simulink model "controller"  (R2020b)
settings: Solver=ode23  StartTime=0.0  StopTime=Tsim  RelTol=1e-3
values from neighbouring files (symbols this model uses):
  pg_traj = create_traj(state_list, Nsamples)    [ctrl_ds_setup.m]
undefined symbols (not defined in the file or in its folder): ctrl_cfg_rem
libraries: biped_lib x2
settings Model: Creator=isclab  LastModifiedBy=isclab
settings SFSimCC: MATLABDynamicMemAlloc=off

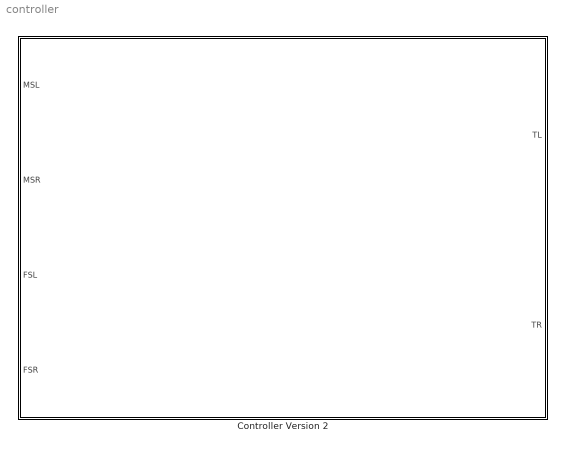
== system controller ==
  Controller Version 2 : Subsystem

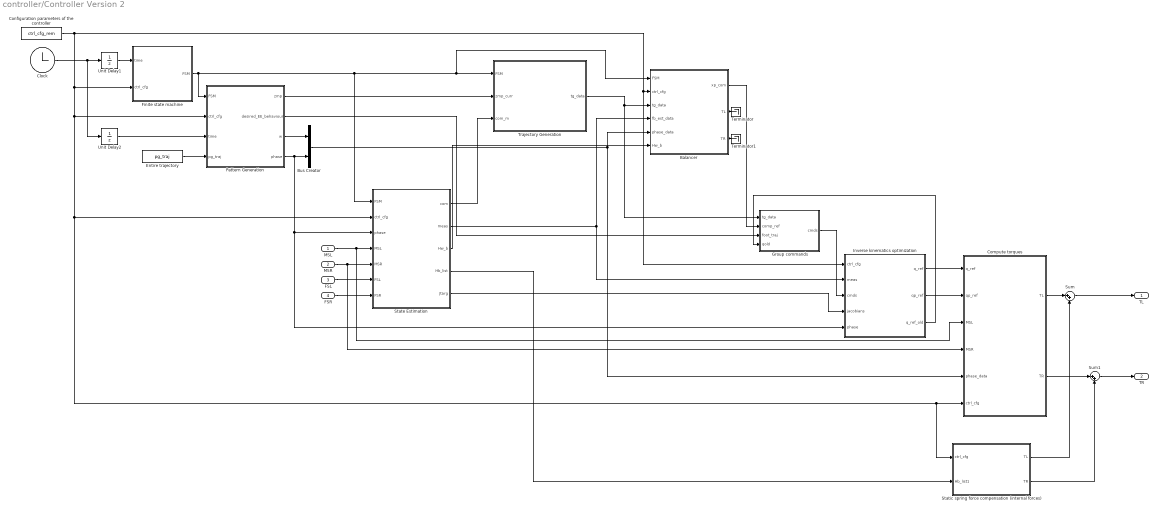
== system controller/Controller Version 2 ==
  MSL : Inport
  MSR : Inport  Port=2
  FSL : Inport  Port=3
  FSR : Inport  Port=4
  Balancer : MATLAB Function  TreatAsAtomicUnit=on
  Bus Creator : BusCreator  Inputs=2
  Clock : Clock
  Compute torques : Subsystem
  Configuration parameters of the controller : Constant  Value=ctrl_cfg_rem  OutDataTypeStr=Bus: ctrl_cfg_rem_bus  SampleTime=ctrl_cfg_rem.par.Ts
  Entire trajectory : Constant  Value=pg_traj  VectorParams1D=off  OutDataTypeStr=Bus: pg_traj_bus  SampleTime=ctrl_cfg_rem.par.Ts
  Finite state machine : MATLAB Function  TreatAsAtomicUnit=on
  Group commands : Subsystem
  Inverse kinematics optimization : Subsystem  Variant=on  mask{ik_opt=ctrl_cfg_rem.ik_opt, Ts=ctrl_cfg_rem.par.Ts}
      mask prompts: ik_opt "Ikine parameters"; Ts "Sampling time"
  Pattern Generation : Subsystem
  State Estimation : Subsystem  mask{fb_est=ctrl_cfg_rem.fb_est, Ts=ctrl_cfg_rem.par.Ts}
      mask prompts: fb_est "Floating base est. params"; Ts "Sampling time"
  Static spring force compensation (internal forces) : Subsystem
  Sum : Sum  Inputs=|++
  Sum1 : Sum  Inputs=|++
  Terminator : Terminator
  Terminator1 : Terminator
  Trajectory Generation : Subsystem  Variant=on  mask{tg=ctrl_cfg_rem.tg}
      mask prompts: tg "Preview controller parameters"
  Unit Delay1 : UnitDelay  SampleTime=ctrl_cfg_rem.par.Ts  HasFrameUpgradeWarning=on
  Unit Delay2 : UnitDelay  SampleTime=ctrl_cfg_rem.par.Ts  HasFrameUpgradeWarning=on
  TL : Outport
  TR : Outport  Port=2
  wires:
  Pattern Generation/1(zmp) -> Trajectory Generation/2(zmp_curr)
  Pattern Generation/4(phase) -> State Estimation/3(phase), Inverse kinematics optimization/5(phase), Bus Creator/2
  Unit Delay1/1 -> Finite state machine/1(time)
  Clock/1 -> Unit Delay2/1, Unit Delay1/1
  MSL/1 -> State Estimation/4(MSL), Compute torques/3(MSL)
  Entire trajectory/1 -> Pattern Generation/4(pg_traj)
  MSR/1 -> State Estimation/5(MSR), Compute torques/4(MSR)
  FSR/1 -> State Estimation/7(FSR)
  Configuration parameters of the controller/1 -> Inverse kinematics optimization/1(ctrl_cfg), Balancer/2(ctrl_cfg), Static spring force compensation (internal forces)/1(ctrl_cfg), Compute torques/6(ctrl_cfg), State Estimation/2(ctrl_cfg), Pattern Generation/2(ctrl_cfg), Finite state machine/2(ctrl_cfg)
  Finite state machine/1(FSM) -> Pattern Generation/1(FSM), State Estimation/1(FSM), Balancer/1(FSM), Trajectory Generation/1(FSM)
  Unit Delay2/1 -> Pattern Generation/3(time)
  FSL/1 -> State Estimation/6(FSL)
  Pattern Generation/3(w) -> Bus Creator/1
  Balancer/2(TL) -> Terminator/1
  Balancer/3(TR) -> Terminator1/1
  Bus Creator/1 -> Compute torques/5(phase_data), Balancer/5(phase_data)
  Inverse kinematics optimization/1(q_ref) -> Compute torques/1(q_ref)
  Inverse kinematics optimization/2(qp_ref) -> Compute torques/2(qp_ref)
  State Estimation/5(Jtarg) -> Inverse kinematics optimization/4(jacobians)
  Compute torques/1(TL) -> Sum/1
  Sum/1 -> TL/1
  Sum1/1 -> TR/1
  Compute torques/2(TR) -> Sum1/1
  State Estimation/4(Hb_list) -> Static spring force compensation (internal forces)/2(Hb_list1)
  Static spring force compensation (internal forces)/1(TL) -> Sum/2
  Static spring force compensation (internal forces)/2(TR) -> Sum1/2
  State Estimation/1(com) -> Trajectory Generation/3(com_m)
  State Estimation/2(meas) -> Inverse kinematics optimization/2(meas), Balancer/4(fb_est_data)
  Trajectory Generation/1(tg_data) -> Balancer/3(tg_data), Group commands/1(tg_data)
  Balancer/1(xp_com) -> Group commands/2(comp_ref)
  Pattern Generation/2(desired_EE_behaviour) -> Group commands/3(foot_traj)
  Group commands/1(cmds) -> Inverse kinematics optimization/3(cmds)
  State Estimation/3(Hw_b) -> Balancer/6(Hw_b)
  Inverse kinematics optimization/3(q_ref_old) -> Group commands/4(qold)

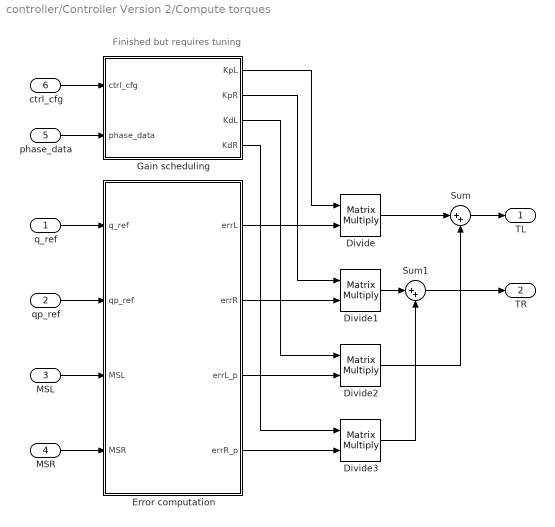
== system controller/Controller Version 2/Compute torques ==
  note: Finished but requires tuning
  q_ref : Inport
  qp_ref : Inport  Port=2
  MSL : Inport  Port=3
  MSR : Inport  Port=4
  phase_data : Inport  Port=5
  ctrl_cfg : Inport  Port=6
  Divide{,1..3} (4 alike) : Product  Inputs=**  Multiplication=Matrix(*)
  Error computation : MATLAB Function  TreatAsAtomicUnit=on
  Gain scheduling : MATLAB Function  TreatAsAtomicUnit=on
  Sum : Sum  Inputs=|++
  Sum1 : Sum  Inputs=|++
  TL : Outport
  TR : Outport  Port=2
  wires:
  phase_data/1 -> Gain scheduling/2(phase_data)
  MSL/1 -> Error computation/3(MSL)
  MSR/1 -> Error computation/4(MSR)
  qp_ref/1 -> Error computation/2(qp_ref)
  q_ref/1 -> Error computation/1(q_ref)
  Gain scheduling/1(KpL) -> Divide/1
  Error computation/1(errL) -> Divide/2
  Error computation/2(errR) -> Divide1/2
  Error computation/4(errR_p) -> Divide3/2
  Error computation/3(errL_p) -> Divide2/2
  Divide/1 -> Sum/1
  Divide2/1 -> Sum/2
  Sum/1 -> TL/1
  Divide1/1 -> Sum1/1
  Divide3/1 -> Sum1/2
  Sum1/1 -> TR/1
  ctrl_cfg/1 -> Gain scheduling/1(ctrl_cfg)
  Gain scheduling/2(KpR) -> Divide1/1
  Gain scheduling/3(KdL) -> Divide2/1
  Gain scheduling/4(KdR) -> Divide3/1

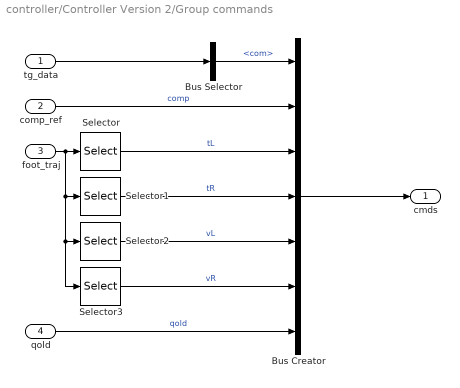
== system controller/Controller Version 2/Group commands ==
  tg_data : Inport
  comp_ref : Inport  Port=2
  foot_traj : Inport  Port=3
  qold : Inport  Port=4
  Bus Creator : BusCreator  Inputs=7
  Bus Selector : BusSelector  OutputSignals=com
  Selector : Selector  InputPortWidth=12  IndexOptions=Index vector (dialog)  Indices=[1:3]  OutputSizes=1
  Selector1 : Selector  InputPortWidth=12  IndexOptions=Index vector (dialog)  Indices=[4:6]  OutputSizes=1
  Selector2 : Selector  InputPortWidth=12  IndexOptions=Index vector (dialog)  Indices=[7:9]  OutputSizes=1
  Selector3 : Selector  InputPortWidth=12  IndexOptions=Index vector (dialog)  Indices=[10:12]  OutputSizes=1
  cmds : Outport
  wires:
  Bus Creator/1 -> cmds/1
  comp_ref/1 -> Bus Creator/2  "comp"
  tg_data/1 -> Bus Selector/1
  qold/1 -> Bus Creator/7  "qold"
  Bus Selector/1 -> Bus Creator/1  "<com>"
  foot_traj/1 -> Selector3/1, Selector2/1, Selector1/1, Selector/1
  Selector/1 -> Bus Creator/3  "tL"
  Selector1/1 -> Bus Creator/4  "tR"
  Selector2/1 -> Bus Creator/5  "vL"
  Selector3/1 -> Bus Creator/6  "vR"

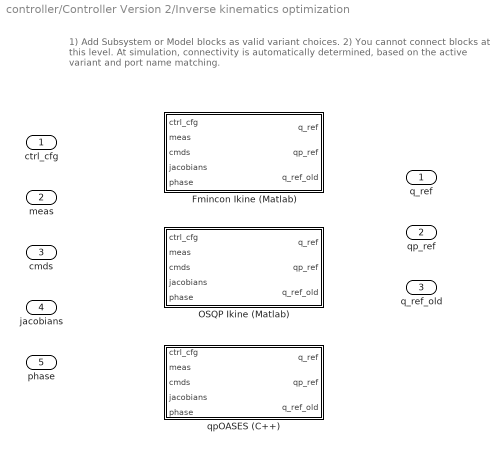
== system controller/Controller Version 2/Inverse kinematics optimization ==
  note: 1) Add Subsystem or Model blocks as valid variant choices.
      | 2) You cannot connect blocks at this level. At simulation, connectivity is automatically
      | determined, based on the active variant and port name matching.
  ctrl_cfg : Inport
  meas : Inport  Port=2
  cmds : Inport  Port=3
  jacobians : Inport  Port=4
  phase : Inport  Port=5
  Fmincon Ikine (Matlab) : Subsystem  VariantControl=VAR_IK ==1
  OSQP Ikine (Matlab) : Subsystem  VariantControl=VAR_IK ==2
  qpOASES (C++) : Subsystem  VariantControl=VAR_IK ==3
  q_ref : Outport
  qp_ref : Outport  Port=2
  q_ref_old : Outport  Port=3

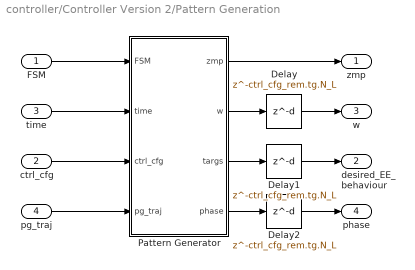
== system controller/Controller Version 2/Pattern Generation ==
  FSM : Inport
  ctrl_cfg : Inport  Port=2
  time : Inport  Port=3
  pg_traj : Inport  Port=4
  Delay : Delay  DelayLength=ctrl_cfg_rem.tg.N_L  InitialCondition=0  SampleTime=ctrl_cfg_rem.par.Ts
  Delay1 : Delay  DelayLength=ctrl_cfg_rem.tg.N_L  InitialCondition=0  SampleTime=ctrl_cfg_rem.par.Ts
  Delay2 : Delay  DelayLength=ctrl_cfg_rem.tg.N_L  InitialCondition=0  SampleTime=ctrl_cfg_rem.par.Ts
  Pattern Generator : MATLAB Function  TreatAsAtomicUnit=on
  zmp : Outport
  desired_EE_behaviour : Outport  Port=2
  w : Outport  Port=3
  phase : Outport  Port=4
  wires:
  Delay1/1 -> desired_EE_behaviour/1
  time/1 -> Pattern Generator/2(time)
  pg_traj/1 -> Pattern Generator/4(pg_traj)
  Delay/1 -> w/1
  FSM/1 -> Pattern Generator/1(FSM)
  Pattern Generator/1(zmp) -> zmp/1
  Pattern Generator/2(w) -> Delay/1
  ctrl_cfg/1 -> Pattern Generator/3(ctrl_cfg)
  Delay2/1 -> phase/1
  Pattern Generator/4(phase) -> Delay2/1
  Pattern Generator/3(targs) -> Delay1/1

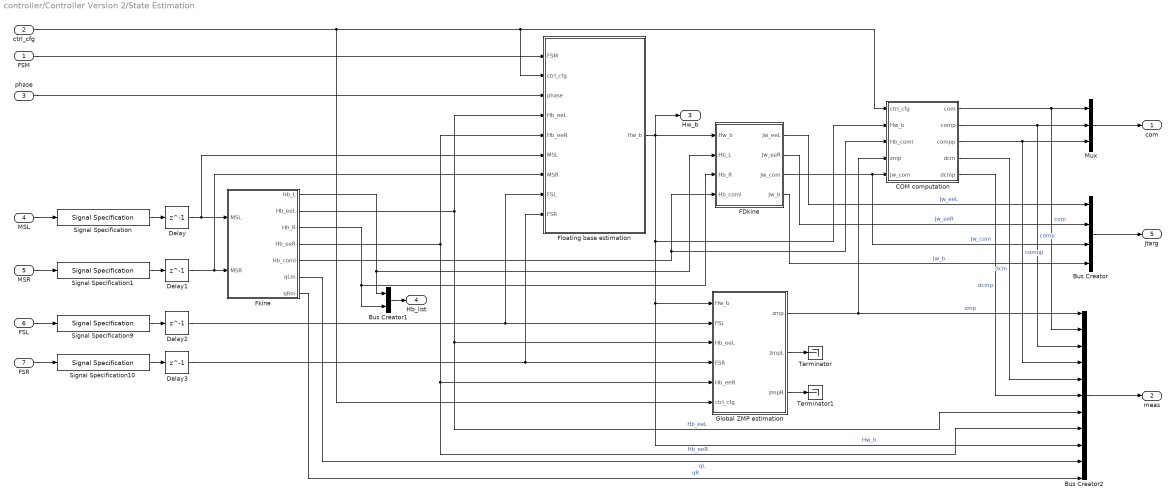
== system controller/Controller Version 2/State Estimation ==
  FSM : Inport
  ctrl_cfg : Inport  Port=2
  phase : Inport  Port=3
  MSL : Inport  Port=4
  MSR : Inport  Port=5
  FSL : Inport  Port=6
  FSR : Inport  Port=7
  Bus Creator : BusCreator  Inputs=4
  Bus Creator1 : BusCreator  Inputs=2
  Bus Creator2 : BusCreator  Inputs=11
  COM computation : MATLAB Function  TreatAsAtomicUnit=on
  Delay : Delay  DelayLength=1  InitialCondition=fb_est.init.MSL  SampleTime=Ts
  Delay1 : Delay  DelayLength=1  InitialCondition=fb_est.init.MSR  SampleTime=Ts
  Delay2 : Delay  DelayLength=1  InitialCondition=fb_est.init.FSL  SampleTime=Ts
  Delay3 : Delay  DelayLength=1  InitialCondition=fb_est.init.FSR  SampleTime=Ts
  FDkine : MATLAB Function  TreatAsAtomicUnit=on
  Fkine : MATLAB Function  TreatAsAtomicUnit=on
  Floating base estimation : MATLAB Function  TreatAsAtomicUnit=on
  Global ZMP estimation : MATLAB Function  TreatAsAtomicUnit=on
  Mux : Mux  Inputs=3
  Signal Specification : SignalSpecification  OutDataTypeStr=Bus: leg_str_bus
  Signal Specification1 : SignalSpecification  OutDataTypeStr=Bus: leg_str_bus
  Signal Specification10 : SignalSpecification  OutDataTypeStr=Bus: fs_str_bus
  Signal Specification9 : SignalSpecification  OutDataTypeStr=Bus: fs_str_bus
  Terminator : Terminator
  Terminator1 : Terminator
  com : Outport
  meas : Outport  Port=2
  Hw_b : Outport  Port=3
  Hb_list : Outport  Port=4
  Jtarg : Outport  Port=5
  wires:
  Signal Specification/1 -> Delay/1
  Signal Specification1/1 -> Delay1/1
  Signal Specification9/1 -> Delay2/1
  Signal Specification10/1 -> Delay3/1
  Delay2/1 -> Global ZMP estimation/2(FSL), Floating base estimation/8(FSL)
  Delay3/1 -> Global ZMP estimation/4(FSR), Floating base estimation/9(FSR)
  Fkine/1(Hb_L) -> Bus Creator1/1, FDkine/2(Hb_L)
  Fkine/3(Hb_R) -> Bus Creator1/2, FDkine/3(Hb_R)
  phase/1 -> Floating base estimation/3(phase)
  FSM/1 -> Floating base estimation/1(FSM)
  Floating base estimation/1(Hw_b) -> Hw_b/1, Bus Creator2/9, Global ZMP estimation/1(Hw_b), COM computation/2(Hw_b), FDkine/1(Hw_b)  "Hw_b"
  Fkine/5(Hb_comi) -> FDkine/4(Hb_comi), COM computation/3(Hb_comi)
  FDkine/3(Jw_com) -> COM computation/5(Jw_com), Bus Creator/3  "Jw_com"
  FDkine/1(Jw_eeL) -> Bus Creator/1  "Jw_eeL"
  FDkine/2(Jw_eeR) -> Bus Creator/2  "Jw_eeR"
  FDkine/4(Jw_b) -> Bus Creator/4  "Jw_b"
  Bus Creator/1 -> Jtarg/1
  ctrl_cfg/1 -> Global ZMP estimation/6(ctrl_cfg), COM computation/1(ctrl_cfg), Floating base estimation/2(ctrl_cfg)
  Global ZMP estimation/1(zmp) -> Bus Creator2/1, COM computation/4(zmp)  "zmp"
  Delay/1 -> Floating base estimation/6(MSL), Fkine/1(MSL)
  Delay1/1 -> Floating base estimation/7(MSR), Fkine/2(MSR)
  MSL/1 -> Signal Specification/1
  MSR/1 -> Signal Specification1/1
  FSL/1 -> Signal Specification9/1
  FSR/1 -> Signal Specification10/1
  Global ZMP estimation/2(zmpL) -> Terminator/1
  Global ZMP estimation/3(zmpR) -> Terminator1/1
  Bus Creator1/1 -> Hb_list/1
  COM computation/1(com) -> Mux/1, Bus Creator2/2  "com"
  COM computation/2(comp) -> Mux/2, Bus Creator2/3  "comp"
  COM computation/3(compp) -> Mux/3, Bus Creator2/4  "compp"
  COM computation/4(dcm) -> Bus Creator2/5  "dcm"
  COM computation/5(dcmp) -> Bus Creator2/6  "dcmp"
  Fkine/2(Hb_eeL) -> Floating base estimation/4(Hb_eeL), Global ZMP estimation/3(Hb_eeL), Bus Creator2/7  "Hb_eeL"
  Fkine/4(Hb_eeR) -> Floating base estimation/5(Hb_eeR), Global ZMP estimation/5(Hb_eeR), Bus Creator2/8  "Hb_eeR"
  Fkine/6(qLm) -> Bus Creator2/10  "qL"
  Fkine/7(qRm) -> Bus Creator2/11  "qR"
  Bus Creator2/1 -> meas/1
  Mux/1 -> com/1

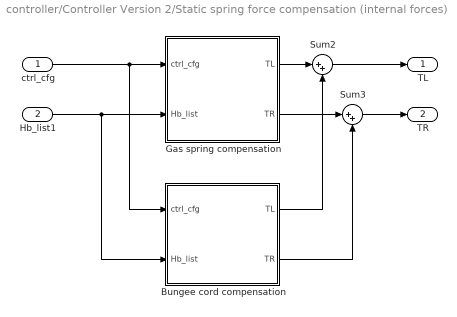
== system controller/Controller Version 2/Static spring force compensation (internal forces) ==
  ctrl_cfg : Inport
  Hb_list1 : Inport  Port=2
  Bungee cord compensation : MATLAB Function  TreatAsAtomicUnit=on
  Gas spring compensation : MATLAB Function  TreatAsAtomicUnit=on
  Sum2 : Sum  Inputs=|++
  Sum3 : Sum  Inputs=|++
  TL : Outport
  TR : Outport  Port=2
  wires:
  Bungee cord compensation/1(TL) -> Sum2/2
  Sum2/1 -> TL/1
  Sum3/1 -> TR/1
  Bungee cord compensation/2(TR) -> Sum3/2
  ctrl_cfg/1 -> Bungee cord compensation/1(ctrl_cfg), Gas spring compensation/1(ctrl_cfg)
  Hb_list1/1 -> Bungee cord compensation/2(Hb_list), Gas spring compensation/2(Hb_list)
  Gas spring compensation/1(TL) -> Sum2/1
  Gas spring compensation/2(TR) -> Sum3/1

== system controller/Controller Version 2/Trajectory Generation ==
  note: 1) Add Subsystem or Model blocks as valid variant choices.
      | 2) You cannot connect blocks at this level. At simulation, connectivity is automatically
      | determined, based on the active variant and port name matching.
  FSM : Inport
  zmp_curr : Inport  Port=2
  com_m : Inport  Port=3
  (C++ impl) : Subsystem  VariantControl=VAR_TG == 2
  Preview Controller (simulink impl) : Subsystem  VariantControl=VAR_TG == 1
  tg_data : Outport

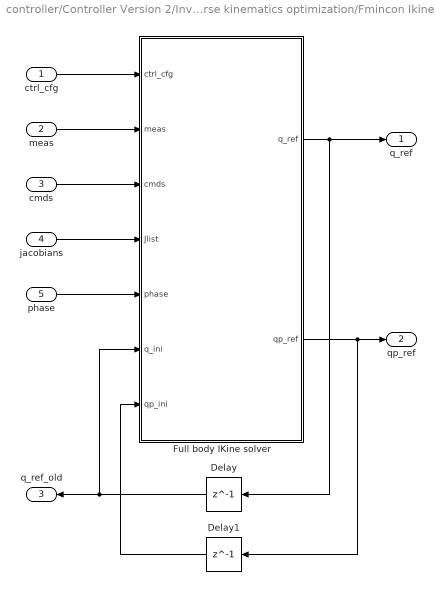
== system controller/Controller Version 2/Inverse kinematics optimization/Fmincon Ikine (Matlab) ==
  ctrl_cfg : Inport
  meas : Inport  Port=2
  cmds : Inport  Port=3
  jacobians : Inport  Port=4
  phase : Inport  Port=5
  Delay : Delay  DelayLength=1  InitialCondition=ik_opt.q_ini  SampleTime=Ts
  Delay1 : Delay  DelayLength=1  InitialCondition=ik_opt.qp_ini  SampleTime=Ts
  Full body IKine solver : MATLAB Function  TreatAsAtomicUnit=on
  q_ref : Outport
  qp_ref : Outport  Port=2
  q_ref_old : Outport  Port=3
  wires:
  Full body IKine solver/2(qp_ref) -> Delay1/1, qp_ref/1
  Full body IKine solver/1(q_ref) -> Delay/1, q_ref/1
  meas/1 -> Full body IKine solver/2(meas)
  cmds/1 -> Full body IKine solver/3(cmds)
  phase/1 -> Full body IKine solver/5(phase)
  jacobians/1 -> Full body IKine solver/4(Jlist)
  Delay/1 -> q_ref_old/1, Full body IKine solver/6(q_ini)
  Delay1/1 -> Full body IKine solver/7(qp_ini)
  ctrl_cfg/1 -> Full body IKine solver/1(ctrl_cfg)

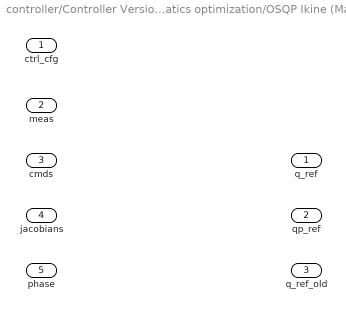
== system controller/Controller Version 2/Inverse kinematics optimization/OSQP Ikine (Matlab) ==
  ctrl_cfg : Inport
  meas : Inport  Port=2
  cmds : Inport  Port=3
  jacobians : Inport  Port=4
  phase : Inport  Port=5
  q_ref : Outport
  qp_ref : Outport  Port=2
  q_ref_old : Outport  Port=3

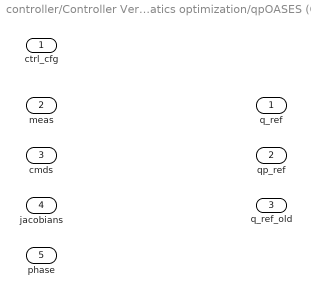
== system controller/Controller Version 2/Inverse kinematics optimization/qpOASES (C++) ==
  ctrl_cfg : Inport
  meas : Inport  Port=2
  cmds : Inport  Port=3
  jacobians : Inport  Port=4
  phase : Inport  Port=5
  q_ref : Outport
  qp_ref : Outport  Port=2
  q_ref_old : Outport  Port=3

== system controller/Controller Version 2/Trajectory Generation/(C++ impl) ==
  FSM : Inport
  zmp_curr : Inport  Port=2
  com_m : Inport  Port=3
  tg_data : Outport

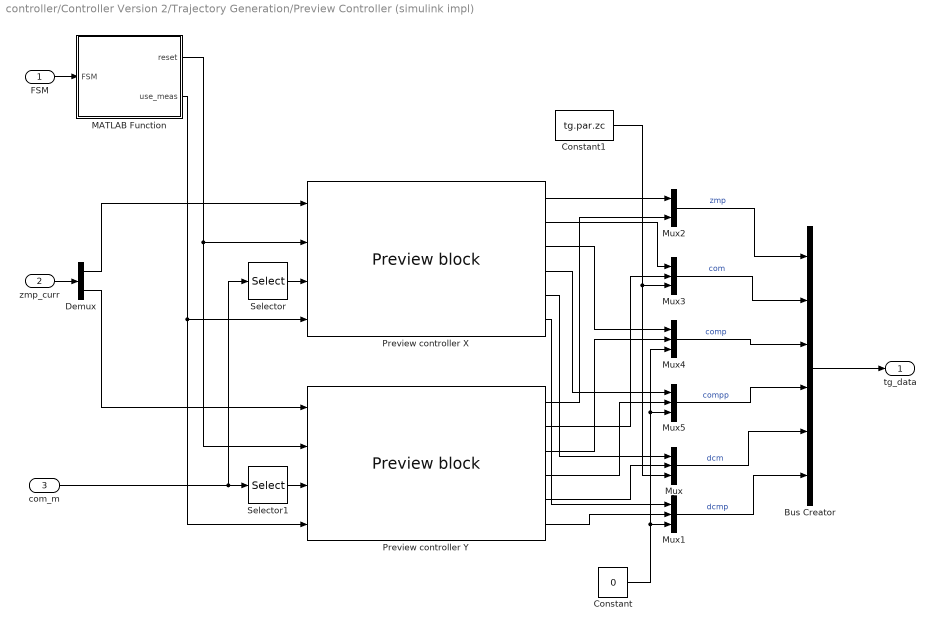
== system controller/Controller Version 2/Trajectory Generation/Preview Controller (simulink impl) ==
  FSM : Inport
  zmp_curr : Inport  Port=2
  com_m : Inport  Port=3
  Bus Creator : BusCreator  Inputs=6
  Constant : Constant  Value=0
  Constant1 : Constant  Value=tg.par.zc
  Demux : Demux  Outputs=2
  MATLAB Function : MATLAB Function  TreatAsAtomicUnit=on
  Mux{,1,3..5} (5 alike) : Mux  Inputs=3
  Mux2 : Mux  Inputs=2
  Preview controller X : biped_lib/Preview block  Pctrl=tg
  Preview controller Y : biped_lib/Preview block  Pctrl=tg
  Selector : Selector  InputPortWidth=6  IndexOptions=Index vector (dialog)  Indices=[1:3]  OutputSizes=1
  Selector1 : Selector  InputPortWidth=6  IndexOptions=Index vector (dialog)  Indices=[4:6]  OutputSizes=1
  tg_data : Outport
  wires:
  zmp_curr/1 -> Demux/1
  Demux/1 -> Preview controller X/1
  Demux/2 -> Preview controller Y/1
  com_m/1 -> Selector/1, Selector1/1
  Selector/1 -> Preview controller X/3
  Selector1/1 -> Preview controller Y/3
  FSM/1 -> MATLAB Function/1(FSM)
  MATLAB Function/1(reset) -> Preview controller X/2, Preview controller Y/2
  MATLAB Function/2(use_meas) -> Preview controller Y/4, Preview controller X/4
  Preview controller Y/5 -> Mux/2
  Preview controller Y/6 -> Mux1/2
  Preview controller X/5 -> Mux/1
  Preview controller X/6 -> Mux1/1
  Preview controller X/1 -> Mux2/1
  Preview controller Y/1 -> Mux2/2
  Mux2/1 -> Bus Creator/1  "zmp"
  Mux/1 -> Bus Creator/5  "dcm"
  Mux1/1 -> Bus Creator/6  "dcmp"
  Preview controller X/2 -> Mux3/1
  Preview controller Y/2 -> Mux3/2
  Mux3/1 -> Bus Creator/2  "com"
  Mux4/1 -> Bus Creator/3  "comp"
  Preview controller X/3 -> Mux4/1
  Preview controller Y/3 -> Mux4/2
  Mux5/1 -> Bus Creator/4  "compp"
  Preview controller X/4 -> Mux5/1
  Preview controller Y/4 -> Mux5/2
  Constant/1 -> Mux4/3, Mux5/3, Mux1/3
  Constant1/1 -> Mux3/3, Mux/3
  Bus Creator/1 -> tg_data/1

== matlab function controller/Controller Version 2/State Estimation/COM computation ==
  data: ctrl_cfg input; Hw_b input; Hb_comi input; zmp input; com output; comp output; compp output; dcm output; Jw_com input; dcmp output
function [com, comp, compp, dcm, dcmp] = fcn(ctrl_cfg, Hw_b, Hb_comi, zmp, Jw_com)
persistent init com_old comp_old compp_old;

fb_est = ctrl_cfg.fb_est;
Ts = fb_est.Ts;
omega = fb_est.omega;
mlist = fb_est.mlist;

% IIR filter parameters
alpha_cp = fb_est.alpha_cp;
alpha_cpp = fb_est.alpha_cpp;

if isempty(init)
    init = 1;
    com_old = fb_est.init.com; %prevents controller jumps
    comp_old = zeros(3,1);
    compp_old = zeros(3,1);
end

% compute com position in base frame
com_b = compute_com_pos(Hb_comi,mlist);

% get estimated com postion
com_w = Hw_b * [com_b;1];

% compute com outputs
com = com_w(1:3);
comp = alpha_cp*(com-com_old)/Ts + (1-alpha_cp)*comp_old;
compp = alpha_cpp*(comp-com_old)/Ts + (1-alpha_cpp)*compp_old;

% there is a possible way of computing the velocity using other data
% sources as well. Try it out if there is enough time.

% overwrite old values
com_old = com;
comp_old = comp;
compp_old = compp;

% compute dcm outputs
dcm = com + comp/omega;
dcmp = omega * (dcm - zmp);
dcmp_alt = comp + compp/omega; %alternative way of computing dcmp (lag version)

dcm_m = [dcm;dcmp];

== matlab function controller/Controller Version 2/State Estimation/Global ZMP estimation ==
  data: Hw_b input; zmp output; FSL input; Hb_eeL input; FSR input; Hb_eeR input; zmpL output; zmpR output; ctrl_cfg input
function [zmp,zmpL,zmpR] = fcn(Hw_b, FSL,Hb_eeL, FSR, Hb_eeR, ctrl_cfg)
    Hw_eeL = Hw_b * Hb_eeL;
    Hw_eeR = Hw_b * Hb_eeR;

    foot_data = ctrl_cfg.fb_est.foot_data;
    threshold_force = 1;
    simple_zmp = 0;
    [zmp,zmpL_full,zmpR_full] = compute_zmp_full(FSL, FSR, foot_data, Hw_eeL, Hw_eeR, threshold_force, simple_zmp); %computed zmp
    zmpL = zmpL_full.glo;
    zmpR = zmpR_full.glo;
end

== matlab function controller/Controller Version 2/Static spring force compensation (internal forces)/Bungee cord compensation ==
  data: ctrl_cfg input; Hb_list input; TL output; TR output
function [TL, TR] = fcn(ctrl_cfg, Hb_list)
    consts = ctrl_cfg.sf_comp.bc;
    HL = Hb_list.HL;
    HR = Hb_list.HR;
    [TL, TR] = bcordCompensTorques2(HL,HR,consts);
end

== matlab function controller/Controller Version 2/Compute torques/Gain scheduling ==
  data: ctrl_cfg input; phase_data input; KpL output; KpR output; KdL output; KdR output
function [KpL,KpR,KdL,KdR] = fcn(ctrl_cfg,phase_data)
    test_type = ctrl_cfg.fsm.test_type;
    w = phase_data.w;
    WshiftL = w(1);
    WshiftR = w(2);
    phase = phase_data.phase;
    [KpL, KpR, KdL, KdR] = get_gains2(test_type, phase, WshiftL, WshiftR);
end

== matlab function controller/Controller Version 2/Compute torques/Error computation ==
  data: q_ref input; qp_ref input; MSL input; errL output; MSR input; errR output; errL_p output; errR_p output
function [errL, errR, errL_p, errR_p] = fcn(q_ref, qp_ref, MSL, MSR)
% reference positions
qL_ref = q_ref(1:end/2);
qR_ref = q_ref(end/2+1:end);
% reference velocities
qLp_ref = qp_ref(1:end/2);
qRp_ref = qp_ref(end/2+1:end);

% measurement data
[LL,RL] = group_motor_data(MSL,MSR);
% measured positions
qL_m = LL.q;
qR_m = RL.q;
% measured velocities
qLp_m = LL.qp;
qRp_m = RL.qp;

% position errors
errL = qL_ref-qL_m;
errR = qR_ref-qR_m;

% velocity errors
errL_p = qLp_ref-qLp_m;
errR_p = qRp_ref-qRp_m;

== matlab function controller/Controller Version 2/Inverse kinematics optimization/Fmincon Ikine (Matlab)/Full body IKine solver ==
  data: ctrl_cfg input; meas input; q_ref output; cmds input; Jlist input; phase input; qp_ref output; q_ini input; qp_ini input
function [q_ref,qp_ref] = fcn(ctrl_cfg, meas, cmds, Jlist, phase, q_ini, qp_ini)
[q_ref,qp_ref] = ikine_step2(meas, cmds, q_ini, qp_ini, Jlist, ctrl_cfg);

== matlab function controller/Controller Version 2/Finite state machine ==
  data: time input; FSM output Bus: FSM_bus; ctrl_cfg input
function FSM = fcn(time, ctrl_cfg)

test_type = ctrl_cfg.fsm.test_type;
Tpause = ctrl_cfg.fsm.Tpause;

FSM = fsm_ctrl_struct;

% wait for the fb estimation to get the correct state
if time > Tpause
    FSM.bal.act = 1;
    if test_type ~= 0
        FSM.pg_act = 1;
        FSM.tg.act = 1;
    end
end

== matlab function controller/Controller Version 2/Pattern Generation/Pattern Generator ==
  data: FSM input; zmp output; time input; ctrl_cfg input; w output; targs output; phase output; pg_traj input
function [zmp,w,targs,phase]  = fcn(FSM, time, ctrl_cfg, pg_traj)
persistent t0;

traj = pg_traj;
Ts = ctrl_cfg.par.Ts;

if isempty(t0)
    t0 = time;
end

if ~FSM.pg_act
    %reset the time
    t0 = time;
    %output the zero values
    zmp = traj.zmp(:,1);
    w = traj.w(:,1);
    targs = [
        traj.foot.xL(:,1);
        traj.foot.xR(:,1);
        traj.foot.xLp(:,1);
        traj.foot.xRp(:,1);
    ];
    phase = traj.phase(1);
else
    t1 = time - t0;
    ii = round(t1/Ts);
    zmp = traj.zmp(:,ii);
    w = traj.w(:,ii);
    targs = [
        traj.foot.xL(:,ii);
        traj.foot.xR(:,ii);
        traj.foot.xLp(:,ii);
        traj.foot.xRp(:,ii);
    ];
    phase = traj.phase(ii);
end

== matlab function controller/Controller Version 2/Trajectory Generation/Preview Controller (simulink impl)/MATLAB Function ==
  data: FSM input; reset output; use_meas output
function [reset,use_meas] = fcn(FSM)
% flush buffer memory
if ~FSM.tg.act
    reset = 1;
else
    reset = 0;
end

% use feedback (measured COM)
if FSM.tg.use_fb
    use_meas = 1;
else
    use_meas = 0;
end

== matlab function controller/Controller Version 2/State Estimation/Fkine ==
  data: MSL input; Hb_L output; Hb_eeL output; MSR input; Hb_R output; Hb_eeR output; Hb_comi output; qLm output; qRm output
function [Hb_L, Hb_eeL, Hb_R, Hb_eeR, Hb_comi, qLm, qRm] = fcn(MSL,MSR)
    [LL,RL] = group_motor_data(MSL,MSR);
    qLm = LL.q;
    qRm = RL.q;
    [Hb_comi,Hb_L,Hb_R] = H_com_list(qLm,qRm);
    Hb_eeL = reshape(Hb_L(end,:,:),4,4);
    Hb_eeR = reshape(Hb_R(end,:,:),4,4);
end

== matlab function controller/Controller Version 2/State Estimation/Floating base estimation ==
  data: FSM input; ctrl_cfg input; phase input; Hb_eeL input; Hw_b output; Hb_eeR input; MSL input; MSR input; FSL input; FSR input
function Hw_b = fcn(FSM, ctrl_cfg, phase, Hb_eeL, Hb_eeR, MSL, MSR, FSL, FSR)
    persistent init Hw_L_corr Hw_R_corr;
    persistent quatLimu_old quatRimu_old;
    
    fb_est = ctrl_cfg.fb_est;
    cdf_data = fb_est.cdf_data;
    FootDataPmeas = fb_est.foot_data.fsen.Pmeas;
    
    %begin by not doing any compensation (IMU has no bias yet)
    if isempty(init)
        init = 1;
        %only executed at the init phase
        Hw_eeL = fb_est.init.Hw_eeL;
        Hw_eeR = fb_est.init.Hw_eeR;

        quatLimu_old = [1;0;0;0];
        quatRimu_old = quatLimu_old;
    else
        %if the drift compensation is activated, this is executed every time
        Hw_eeL = Hw_L_corr;
        Hw_eeR = Hw_R_corr;
    end

    %% Measurements from motors
    [LL,RL] = group_motor_data(MSL,MSR);
    aL = LL.a;
    aR = RL.a;
    wL = LL.w;
    wR = RL.w;

    %% IMU based rotation estimation
    %two imu-s that are rigidly attached to the floating base
    R_b_imu1L = rotz(-pi/6);
    R_b_imu1R = rotz(+pi/6);

    %measurements from those two imus
    a1Limu = aL(:,1);
    a1Rimu = aR(:,1);
    w1Limu = wL(:,1);
    w1Rimu = wR(:,1);

    %represent measurements in the base frame (just allignment, not spatial
    %transformation - this means, that we are still working with the
    %acceleration experienced at the position of the IMU)
    a1Lb = R_b_imu1L*a1Limu;
    a1Rb = R_b_imu1R*a1Rimu;
    w1Lb = R_b_imu1R*w1Limu;
    w1Rb = R_b_imu1R*w1Rimu;

    %sampling rate
    dt = fb_est.Ts;
    %use the magdwick algorithm to obtain the estimated rotation in the wcf
    %left
    quatLimu = filter_update(a1Lb, w1Lb, quatLimu_old);
    quatLimu_old = quatLimu;

    %right
    quatRimu = filter_update(a1Rb, w1Rb, quatRimu_old);
    quatRimu_old = quatRimu; 

    %measurements can not be merged directly, as they were obtained in
    %different frames. Calculated quaternions however can be merged, as they
    %are representing the rotation of the same body.
    %averaging rotation matrices - Henze and Ott - documented in 3.2 FB pose
    %est.
    quat_imu_sum = (quatLimu+quatRimu)/2;
    quat_imu_merged = quat_imu_sum/norm(quat_imu_sum); %orientation from the accelerometer
    Rw_b_imu = quat2rotm(quat_imu_merged');

    %% kinematics based rotation estimation
    %translations which are needed for later
    pb_eeL = Hb_eeL(1:3,4);
    pb_eeR = Hb_eeR(1:3,4);

    %kinematic guess for the transformation between wcf and base 
    Hw_b_Lleg = Hw_eeL/Hb_eeL;
    Hw_b_Rleg = Hw_eeR/Hb_eeR;

    %rotations
    Rw_b_Lleg = Hw_b_Lleg(1:3,1:3);
    Rw_b_Rleg = Hw_b_Rleg(1:3,1:3);
    %translations
    pw_b_Lleg = Hw_b_Lleg(1:3,4);
    pw_b_Rleg = Hw_b_Rleg(1:3,4);

    %% fuse all three measurements depending on the leg ZMP measurements
    %flight leg is assigned a low weight, whereas stance leg obtains a high one
    %the closet the zmp is to the edge, the lower the weight is
    zmp_cdf = cdf_data.zmp;
    fcont_cdf = cdf_data.cont;

    %compute the values based on the model and force measurements (LFL&LFR)
    [zmpL] = compute_local_zmp_simple(FSL.Fm,FootDataPmeas);
    [zmpR] = compute_local_zmp_simple(FSR.Fm,FootDataPmeas);
    ftot_L = sum(FSL.Fm);
    ftot_R = sum(FSR.Fm);

    %compute weights
    WL_zmp = max(0,interp2(zmp_cdf.x,zmp_cdf.y,zmp_cdf.p,zmpL(1),zmpL(2)));
    WL_cont = max(0,interp1(fcont_cdf.f,fcont_cdf.p,ftot_L));

    WR_zmp = max(0,interp2(zmp_cdf.x,zmp_cdf.y,zmp_cdf.p,zmpR(2),zmpR(2)));
    WR_cont = max(0,interp1(fcont_cdf.f,fcont_cdf.p,ftot_R));

    %kinematic weights depend on contact estimation and zmp trust region
    WL = WL_zmp*WL_cont;
    WR = WR_zmp*WR_cont;
    Wimu = 0.3;

    eps = 1e-6;
    %normalise weights
    W_norm1 = 1/(WR+WL+eps);
    W_norm2 = 1/(Wimu+WR+WL+eps);
    Wimu_vec = Wimu * [0, W_norm2, W_norm2]; %discard the first angle which is yaw (ZYX convention)
    WL_vec = WL * [W_norm1, W_norm2, W_norm2];
    WR_vec = WR * [W_norm1, W_norm2, W_norm2];

    %fuse measurements using the computed weights
    eul_fused = Wimu_vec.*rotm2eul(Rw_b_imu) + WL_vec.*rotm2eul(Rw_b_Lleg) + WR_vec.*rotm2eul(Rw_b_Rleg);
    Rest_w_b = eul2rotm(eul_fused);

    %% compute the position of the fb in the wcf (averaging two feet)
    pest_w_b = (WL*(Hw_eeL(1:3,4)-Rest_w_b*pb_eeL)+WR*(Hw_eeR(1:3,4)-Rest_w_b*pb_eeR)) * W_norm1;

    %% generate the Hwb transformation and compensate for drifts
    Hest_w_b = [
        Rest_w_b,pest_w_b;
        zeros(1,3),1;
    ];

    %compute drift transformations
    HLdrift = Hw_eeL\Hest_w_b*Hb_eeL;
    HRdrift = Hw_eeR\Hest_w_b*Hb_eeR;

    %compensation factor (between 0 [no convg] and 1 [full comp]) - has to be
    %tuned
    alpha = fb_est.alpha; 
    %it is correct that left and right side are inverted, as stance foot will
    %not drift, however it determines how much the swing foot will
    alphaL = alpha*WR;
    alphaR = alpha*WL;
    [HcorrL,~,~] = transformtraj(eye(4),HLdrift,[0 1],alphaL);
    [HcorrR,~,~] = transformtraj(eye(4),HRdrift,[0 1],alphaR);
    Hw_L_corr = Hw_eeL*HcorrL;
    Hw_R_corr = Hw_eeR*HcorrR;

    Hw_b = Hest_w_b;
end

== matlab function controller/Controller Version 2/Balancer ==
  data: FSM input; ctrl_cfg input; tg_data input; xp_com output; fb_est_data input; TL output; TR output; phase_data input; Hw_b input
function [xp_com,TL,TR] = fcn(FSM, ctrl_cfg, tg_data, fb_est_data, phase_data, Hw_b)
    persistent init dcm_int cz_int v_com_old;
    if isempty(init)
        init = 1;
        dcm_int = zeros(2,1);
        cz_int = 0;
        v_com_old = zeros(3,1);
    end


    %% data about support
    w = phase_data.w;
    WshiftL = w(1);
    WshiftR = w(2);
    phase = phase_data.phase;

    %% constants & configuration
    Ts = ctrl_cfg.par.Ts;
    z_des = ctrl_cfg.bal.com_height;
    g = 9.81;
    omega = sqrt(g/z_des);
    mlist = ctrl_cfg.bal.mlist;
    Mtot = sum(mlist);
    foot_data = ctrl_cfg.bal.foot_data;
    foot_dims = foot_data.dims(1:2)*0.9;
    K = Mtot*omega^2;

    %% read measurements
    zmp_m = fb_est_data.zmp;
    com_m = fb_est_data.com;
    comp_m = fb_est_data.comp;
    dcm_m = fb_est_data.dcm; 

    %% read controls
    zmp_d = tg_data.zmp;
    com_d = tg_data.com;
    comp_d = tg_data.comp;
    dcm_d = tg_data.dcm;
    
    % check if the stabilisation is activated
    if FSM.bal.act
        ctrl_type = 1;
        %% controller possibility 1
        if ctrl_type == 1
            % gains
            Kp_dcm = [1.6*omega;1.3*omega];
            Kp_comz = 1000*omega;
            Kd_comz = 400*omega;
            Ki_comz = 3000*omega;
            Kp_p = [0.2*omega;0.2*omega];
            % leaky integrator
            Ki_dcm = [1*omega;1*omega];
            Kleak = [0.1;0.1];


            % controller
            % com-z
            cz_err = com_d(3) - com_m(3);
            cz_int = cz_int + Ts * cz_err;
            czpp_r = Kd_comz*(comp_d(3)-comp_m(3)) + Kp_comz*cz_err + Ki_comz*cz_int;

            % dcm integrator
            dcm_err = dcm_d(1:2) - dcm_m(1:2); %integral error
            d_err = dcm_err - Kleak.*dcm_int; %inclusion of leakage
            dcm_int = dcm_int + Ts * d_err;

            % reference value for the ZMP
            zmp_r = zmp_d -(1+Kp_dcm./omega).*dcm_err - Ki_dcm./omega.*dcm_int + Kp_p./omega.*(zmp_d-zmp_m);

            % force
            Admittance = eye(3)*0.01;
            Fd = [
                -K*(com_m(1)-zmp_r(1));
                -K*(com_m(2)-zmp_r(2));
                -czpp_r;
            ];

            a_com = Admittance * Fd/Mtot;
            v_com = v_com_old + a_com * Ts; 
            v_com_old = v_com;

        %% controller possibility 2
        elseif ctrl_type == 2

        end
    else
        v_com = zeros(3,1);
    end

    xp_com = v_com;
    TL = zeros(6,1);
    TR = zeros(6,1);

== matlab function controller/Controller Version 2/Static spring force compensation (internal forces)/Gas spring compensation ==
  data: ctrl_cfg input; Hb_list input; TL output; TR output
function [TL, TR] = fcn(ctrl_cfg, Hb_list)
    consts = ctrl_cfg.sf_comp.gs;
    HL = Hb_list.HL;
    HR = Hb_list.HR;
    [TL, TR] = damperCompensTorques2(HL,HR,consts);
end

== matlab function controller/Controller Version 2/State Estimation/FDkine ==
  data: Hw_b input; Jw_eeL output; Hb_L input; Hb_R input; Hb_comi input; Jw_eeR output; Jw_com output; Jw_b output
function [Jw_eeL,Jw_eeR,Jw_com,Jw_b]  = fcn(Hw_b, Hb_L, Hb_R, Hb_comi)
    Hb_i = zeros(Nq+2,4,4); 
    Hb_i(1:end/2,:,:) = Hb_L;
    Hb_i(end/2+1:end,:,:) = Hb_R;

    %% create jacobians
    % get com->base jacobians 
    Jb_comi = compute_com_jac_base(Nq,Hb_i,Hb_comi);

    % get ee->base jaccobian
    Jb_eeL = compute_jacobian(Hb_L,7);
    Jb_eeR = compute_jacobian(Hb_R,7);

    %% transform them to world jacobians and add a jacobian for the base
    frame_flag = 'b';
    % get com->world jacobians 
    Jw_comi = compute_jac_world2(Hw_b,Jb_comi,Hb_i,frame_flag);

    % get ee->world jacobian
    % left
    Hb_eeL = reshape(Hb_L(end,:,:),4,4);
    Jw_eeL_g = compute_jac_world_single2(Hw_b, Jb_eeL, Hb_eeL, 'l', frame_flag);
    % right
    Hb_eeR = reshape(Hb_R(end,:,:),4,4);
    Jw_eeR_g = compute_jac_world_single2(Hw_b, Jb_eeR, Hb_eeR, 'r', frame_flag);

    % get base->world jacobian
    Jw_b_g = compute_jac_world_single2(Hw_b, zeros(6,Nq/2), eye(4), 'b', frame_flag);
    
    %% compute com jacobian
    Jw_com_g = compute_centroidal_jac(Jw_comi,mlist);
    
    %% transform jacobians so that they are consistent with the configuration
    % account for the configuration dependent differences in mapping
    % between generalised and parametrised velocities
    [Efx] = get_FB_matrix(e,Nq,'xyz');

    Jw_eeL = Jw_eeL_g * Efx;
    Jw_eeR = Jw_eeR_g * Efx;
    Jw_b   = Jw_b_g   * Efx;
    Jw_com = Jw_com_g * Efx;
end
